simulink model "soal2"  (R2016b)
settings: Solver=VariableStepAuto  StartTime=0.0  StopTime=100.0  RelTol=1e-3
libraries: fuzblock x1
settings Model: Creator=Mohammad  LastModifiedBy=Mohammad

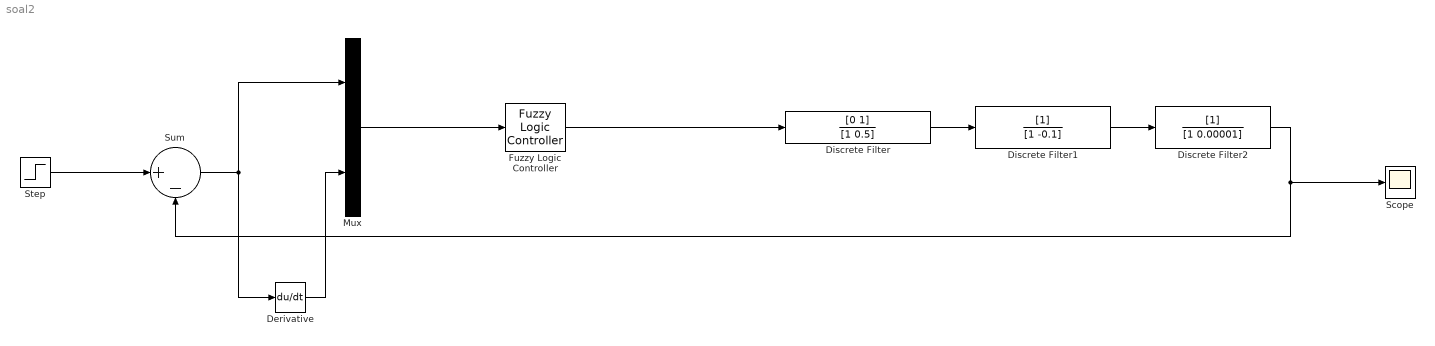
== system soal2 ==
  Derivative : Derivative
  Discrete Filter : DiscreteFilter  Numerator=[0 1]
  Discrete Filter1 : DiscreteFilter  Denominator=[1 -0.1]
  Discrete Filter2 : DiscreteFilter  Denominator=[1 0.00001]
  Fuzzy Logic Controller : fuzblock/Fuzzy Logic  Controller  fis='FKP.fis'
  Mux : Mux  Inputs=2
  Scope : Scope
  Step : Step  SampleTime=0
  Sum : Sum  Inputs=|+-
  wires:
  Discrete Filter/1 -> Discrete Filter1/1
  Discrete Filter1/1 -> Discrete Filter2/1
  Discrete Filter2/1 -> Sum/2, Scope/1
  Step/1 -> Sum/1
  Fuzzy Logic Controller/1 -> Discrete Filter/1
  Mux/1 -> Fuzzy Logic Controller/1
  Derivative/1 -> Mux/2
  Sum/1 -> Mux/1, Derivative/1
